simulink model "test_memristor_vteam_v2_exponential"  (R2018a)
settings: Solver=VariableStepAuto  StartTime=0.0  StopTime=600  FixedStep=1e-4  MaxStep=0.5e-1  MinStep=1e-9  RelTol=1e-3  AbsTol=1e-6
libraries: fl_lib x4, nesl_utility x3, simulink x1
settings Model: Creator=bici  LastModifiedBy=bici
settings SolverCC: InitialStep=1e-9
settings DataIOCC: LimitDataPoints=on  MaxDataPoints=100000  SaveState=on  InspectSignalLogs=on
settings SimscapeCC: SimscapeNormalizeSystem=off

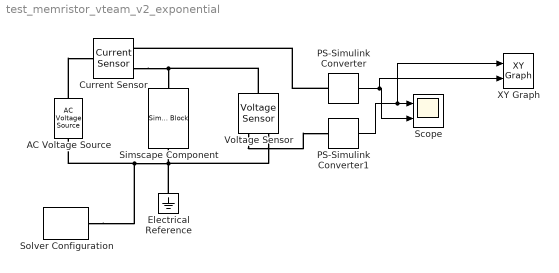
== system test_memristor_vteam_v2_exponential ==
  AC Voltage Source : fl_lib/Electrical/Electrical Sources/AC Voltage Source  amp=0.15 V  shift=0 deg  frequency=1/300 Hz  omega=0 rad/s
  Current Sensor : fl_lib/Electrical/Electrical Sensors/Current Sensor
  Electrical Reference : fl_lib/Electrical/Electrical Elements/Electrical Reference
  PS-Simulink Converter : nesl_utility/PS-Simulink Converter  PhysicalDomain=network_engine_domain  SubClassName=ps_output  LeftPortType=input  RightPortType=output  PseudoPeriodic=off  Frequencies=[]  Unit=1  AffineConversion=off
  PS-Simulink Converter1 : nesl_utility/PS-Simulink Converter  PhysicalDomain=network_engine_domain  SubClassName=ps_output  LeftPortType=input  RightPortType=output  PseudoPeriodic=off  Frequencies=[]  Unit=1  AffineConversion=off
  Scope : Scope  NumInputPorts=2
  Simscape Component : SimscapeComponentBlock  SourceFile=memristor_vteam_v2_exponential  ComponentPath=memristor_vteam_v2_exponential  ComponentVariants=memristor_vteam_v2_exponential  ComponentVariantNames=memristor_vteam_v2_exponential  ClassName=memristor_vteam_v2_exponential  SchemaVersion=1  k_off=5e-4 m/s  v_off=0.145 V  a_off=3  k_on=-1.32e-6 m/s  v_on=-0.09 V  a_on=9  R_off=34 Ohm  w_off=10e-9 m  R_on=17.3 Ohm  w_on=0 m  i_specify=off  i_priority=None  i=0 A  i_nominal_specify=off  i_nominal_unit=A  i_nominal_value=1  v_specify=off  v_priority=None  v=0 V  v_nominal_specify=off  v_nominal_unit=V  v_nominal_value=1
      settings: CopyFcn=simscape.engine.sli.internal.componentblockcallback(gcbh,'COPY')  PreCopyFcn=simscape.engine.sli.internal.componentblockcallback(gcbh,'PRECOPY')  PreDeleteFcn=simscape.engine.sli.internal.componentblockcallback(gcbh,'PREDELETE')
      mask Type: memristor_vteam_v2_exponential
      mask Display:
      | disp('Simscape\n\n\n')
      | disp('\n\n\nmemristor_vteam_v2_exponential');
      | color('red');
      | port_label('RConn', 1,'-');
      | port_label('LConn', 1,'+');
  Solver Configuration : nesl_utility/Solver Configuration  PhysicalDomain=network_engine_domain  SubClassName=solver  LeftPortType=input  RightPortType=generic  Tones=[]  Harmonics=[]  SimulateNoise=off  Profile=off  UseLocalSampling=off  EnableSwitchedLinearOptims=on  FrequencyDomain=off  UseCCode=off  RelTol=0.001  AbsTol=1e-06  MinStep=1e-09  ToWorkspace=off  RevertToSquareIcSolve=off  NumHomotopyIterations=100  PhasorMode=off  PhasorModeNumHarmonics=1  DoDC=off  ResidualTolerance=1e-09  UseLocalSolver=off  LocalSolverChoice=NE_BACKWARD_EULER_ADVANCER  LocalSolverSampleTime=0.001  DoFixedCost=off  MaxNonlinIter=3  MaxModeIter=2  LinearAlgebra=Sparse  EquationFormulation=NE_TIME_EF  DelaysMemoryBudget=1024  AutomaticFiltering=on  FilteringTimeConstant=0.001
  Voltage Sensor : fl_lib/Electrical/Electrical Sensors/Voltage Sensor
  XY Graph : simulink/Sinks/XY Graph  xmin=-0.2  xmax=0.2  ymin=-0.01  ymax=0.01  st=-1
  wires:
  PS-Simulink Converter1/1 -> XY Graph/1, Scope/1
  PS-Simulink Converter/1 -> XY Graph/2, Scope/2
  connections:
  Solver Configuration/RConn1 -- AC Voltage Source/RConn1 -- Voltage Sensor/RConn2 -- Simscape Component/RConn1 -- Electrical Reference/LConn1
  Current Sensor/RConn2 -- Voltage Sensor/LConn1 -- Simscape Component/LConn1
  PS-Simulink Converter/LConn1 -- Current Sensor/RConn1
  Voltage Sensor/RConn1 -- PS-Simulink Converter1/LConn1
  AC Voltage Source/LConn1 -- Current Sensor/LConn1
